simulink model "ex02_model"  (R2023a)
settings: Solver=FixedStepDiscrete  StartTime=0.0  StopTime=0.01  RelTol=1e-3
values from neighbouring files (symbols this model uses):
  a1 = 0.5    [ex02_config.m]
  a2 = -1    [ex02_config.m]
  a3 = 0.5    [ex02_config.m]
  a4 = -1    [ex02_config.m]
  Fc_0 = 1e3    (= 1000)    [ex02_config.m]
  Fc_1 = 4e3    (= 4000)    [ex02_config.m]
  Ts = 1/Fs    (= 6.25e-05)    [ex02_config.m]
libraries: dspsrcs4 x2
settings Model: Creator=daniele  LastModifiedBy=daniele
settings SolverCC: AlgebraicLoopSolver=TrustRegion
settings DataIOCC: ReturnWorkspaceOutputs=off
settings DebuggingCC: UnconnectedInputMsg=warning  UnconnectedOutputMsg=warning  UnconnectedLineMsg=warning  ArithmeticOperatorsInVariantConditions=warning
settings ModelReferenceCC: EnableRefExpFcnMdlSchedulingChecks=on
settings SFSimCC: CustomCodeUndefinedFunction=UseInterfaceOnly

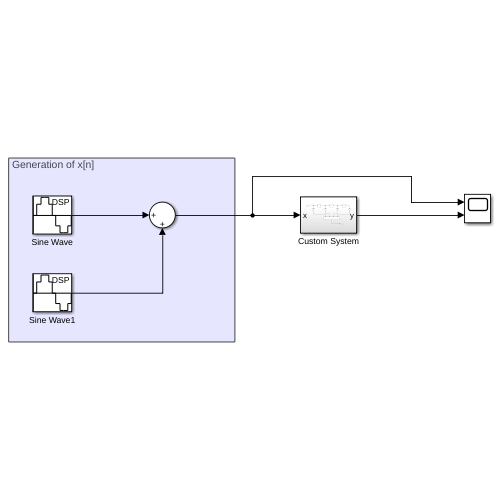
[thumbnail: Simulink's stored preview of the top-level diagram]
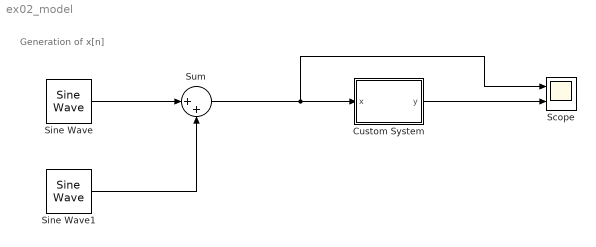
== system ex02_model ==
  note: Generation of x[n]
  Custom System : Subsystem
  Scope : Scope  NumInputPorts=2
  Sine Wave : dspsrcs4/Sine Wave  Amplitude=1  Frequency=Fc_0  Phase=0  SampleMode=Discrete  OutComplex=Complex  CompMethod=Trigonometric fcn  TableSize=Speed  SampleTime=Ts  SamplesPerFrame=1  ResetState=Restart at time zero  OutputFrames=off  dataType=double  wordLen=16  udDataType=sfix(16)  fracBitsMode=Best precision  numFracBits=15  OutDataTypeStr=double  LastOutDataTypeStr=double
  Sine Wave1 : dspsrcs4/Sine Wave  Amplitude=1  Frequency=Fc_1  Phase=0  SampleMode=Discrete  OutComplex=Complex  CompMethod=Trigonometric fcn  TableSize=Speed  SampleTime=Ts  SamplesPerFrame=1  ResetState=Restart at time zero  OutputFrames=off  dataType=double  wordLen=16  udDataType=sfix(16)  fracBitsMode=Best precision  numFracBits=15  OutDataTypeStr=double  LastOutDataTypeStr=double
  Sum : Sum  Inputs=|++
  wires:
  Sine Wave/1 -> Sum/1
  Sine Wave1/1 -> Sum/2
  Sum/1 -> Scope/1, Custom System/1(x)
  Custom System/1(y) -> Scope/2

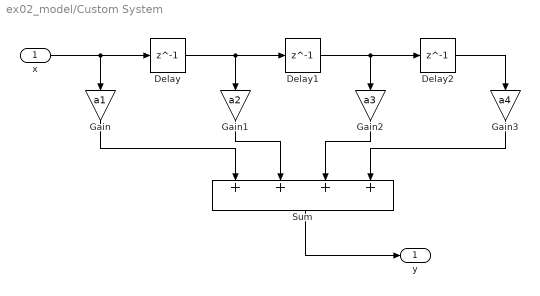
== system ex02_model/Custom System ==
  x : Inport
  Delay : Delay  DelayLength=1
  Delay1 : Delay  DelayLength=1
  Delay2 : Delay  DelayLength=1
  Gain : Gain  Gain=a1
  Gain1 : Gain  Gain=a2
  Gain2 : Gain  Gain=a3
  Gain3 : Gain  Gain=a4
  Sum : Sum  Inputs=++++
  y : Outport
  wires:
  Delay/1 -> Gain1/1, Delay1/1
  x/1 -> Delay/1, Gain/1
  Delay1/1 -> Delay2/1, Gain2/1
  Delay2/1 -> Gain3/1
  Gain1/1 -> Sum/2
  Gain2/1 -> Sum/3
  Gain/1 -> Sum/1
  Gain3/1 -> Sum/4
  Sum/1 -> y/1
